simulink model "controlGPI_pos_2dof_sinMI"  (R2023b)
settings: Solver=ode45  StartTime=0.0  StopTime=tsim  FixedStep=5e-4  MaxStep=tstep
undefined symbols (not defined in the file): contr_robot_params, ddq, dq, ndof, NN_Bspline_params, NN_RBF_params, nn_select, Pc, q, q0, q_cero, q_eq, robot_params, t_qeq_init, t_tr_init, t_trtr, tau_L, tau_L_mags, tr_muestra, Wc, Zc
libraries: simulink x2
(part 1 of 2)
settings Model: Creator=HP  LastModifiedBy=HP

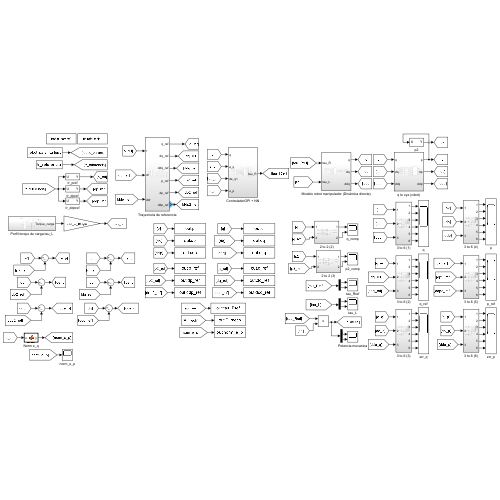
[thumbnail: Simulink's stored preview of the top-level diagram]
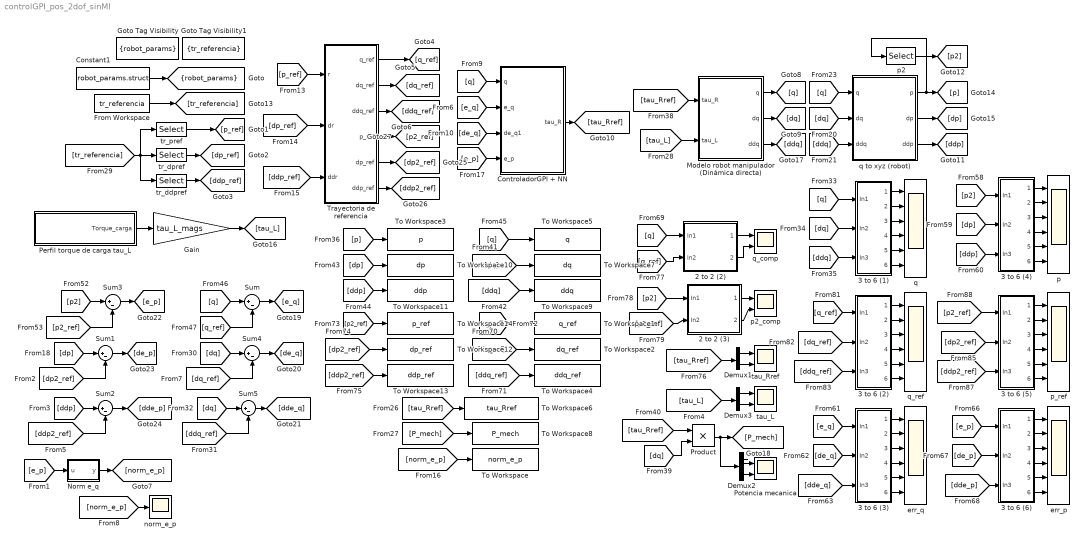
== system controlGPI_pos_2dof_sinMI ==
  2 to 2 (2) : Subsystem
  2 to 2 (3) : Subsystem
  3 to 6 (1) : Subsystem
  3 to 6 (2) : Subsystem
  3 to 6 (3) : Subsystem
  3 to 6 (4) : Subsystem
  3 to 6 (5) : Subsystem
  3 to 6 (6) : Subsystem
  Constant1 : Constant  Value=robot_params.struct  OutDataTypeStr=Bus: robot_params_bus
  ControladorGPI + NN : Subsystem
  Demux1 : Demux  Outputs=2
  Demux2 : Demux  Outputs=2
  Demux3 : Demux  Outputs=2
  From Workspace : FromWorkspace  VariableName=tr_referencia
  Gain : Gain  Gain=tau_L_mags
  Goto Tag Visibility : GotoTagVisibility  GotoTag=robot_params
  Goto Tag Visibility1 : GotoTagVisibility  GotoTag=tr_referencia
  Modelo robot manipulador (Dinámica directa) : Subsystem
  Norm e_q : MATLAB Function  TreatAsAtomicUnit=on
  Perfil torque de carga tau_L : Subsystem
  Potencia mecanica : Scope  NumInputPorts=2
  Product : Product
  Sum{,1..5} (6 alike) : Sum  Inputs=|+-
  To Workspace : ToWorkspace  VariableName=norm_e_p  SaveFormat=Timeseries  SampleTime=-1
  To Workspace1 : ToWorkspace  VariableName=q_ref  SaveFormat=Timeseries  SampleTime=-1
  To Workspace10 : ToWorkspace  VariableName=dp  SaveFormat=Timeseries  SampleTime=-1
  To Workspace11 : ToWorkspace  VariableName=ddp  SaveFormat=Timeseries  SampleTime=-1
  To Workspace12 : ToWorkspace  VariableName=dp_ref  SaveFormat=Timeseries  SampleTime=-1
  To Workspace13 : ToWorkspace  VariableName=ddp_ref  SaveFormat=Timeseries  SampleTime=-1
  To Workspace14 : ToWorkspace  VariableName=p_ref  SaveFormat=Timeseries  SampleTime=-1
  To Workspace2 : ToWorkspace  VariableName=dq_ref  SaveFormat=Timeseries  SampleTime=-1
  To Workspace3 : ToWorkspace  VariableName=p  SaveFormat=Timeseries  SampleTime=-1
  To Workspace4 : ToWorkspace  VariableName=ddq_ref  SaveFormat=Timeseries  SampleTime=-1
  To Workspace5 : ToWorkspace  VariableName=q  SaveFormat=Timeseries  SampleTime=-1
  To Workspace6 : ToWorkspace  VariableName=tau_Rref  SaveFormat=Timeseries  SampleTime=-1
  To Workspace7 : ToWorkspace  VariableName=dq  SaveFormat=Timeseries  SampleTime=-1
  To Workspace8 : ToWorkspace  VariableName=P_mech  SaveFormat=Timeseries  SampleTime=-1
  To Workspace9 : ToWorkspace  VariableName=ddq  SaveFormat=Timeseries  SampleTime=-1
  Trayectoria de referencia : Subsystem
  err_p : Scope  NumInputPorts=6
  err_q : Scope  NumInputPorts=6
  norm_e_p : Scope
  p : Scope  NumInputPorts=6
  p2 : Selector  NumberOfDimensions=2  InputPortWidth=3  IndexOptions=Index vector (dialog),Index vector (dialog)  Indices=[1:2],2  OutputSizes=1,1
  p2_comp : Scope  NumInputPorts=2
  p_ref : Scope  NumInputPorts=6
  q : Scope  NumInputPorts=6
  q to xyz (robot) : Subsystem
  q_comp : Scope  NumInputPorts=2
  q_ref : Scope  NumInputPorts=6
  tau_L : Scope  NumInputPorts=2
  tau_Rref : Scope  NumInputPorts=2
  tr_ddpref : Selector  NumberOfDimensions=2  InputPortWidth=3  IndexOptions=Index vector (dialog),Index vector (dialog)  Indices=[5:6],1  OutputSizes=1,1
  tr_dpref : Selector  NumberOfDimensions=2  InputPortWidth=3  IndexOptions=Index vector (dialog),Index vector (dialog)  Indices=[3:4],1  OutputSizes=1,1
  tr_pref : Selector  NumberOfDimensions=2  InputPortWidth=3  IndexOptions=Index vector (dialog),Index vector (dialog)  Indices=[1:2],1  OutputSizes=1,1
  tag scope: robot_params=scoped
  wires:
  From Workspace/1 -> [tr_referencia]
  Constant1/1 -> [robot_params]
  [tau_L] -> Modelo robot manipulador (Dinámica directa)/2(tau_L)
  [tau_Rref] -> Modelo robot manipulador (Dinámica directa)/1(tau_R)
  Modelo robot manipulador (Dinámica directa)/1(q) -> [q]
  Modelo robot manipulador (Dinámica directa)/2(dq) -> [dq]
  Modelo robot manipulador (Dinámica directa)/3(ddq) -> [ddq]
  ControladorGPI + NN/1(tau_R) -> [tau_Rref]
  [tr_referencia] -> tr_ddpref/1, tr_pref/1, tr_dpref/1
  tr_pref/1 -> [p_ref]
  tr_dpref/1 -> [dp_ref]
  tr_ddpref/1 -> [ddp_ref]
  [e_q] -> 3 to 6 (3)/1(In1)
  [dq_ref] -> 3 to 6 (2)/2(In2)
  [dq] -> 3 to 6 (1)/2(In2)
  2 to 2 (3)/1(1) -> p2_comp/1
  [tau_Rref] -> Product/1
  Product/1 -> Demux2/1, [P_mech]
  [q] -> 3 to 6 (1)/1(In1)
  [p2] -> 2 to 2 (3)/1(In1)
  [ddq_ref] -> 3 to 6 (2)/3(In3)
  3 to 6 (1)/5(Out5) -> q/5
  Demux2/1 -> Potencia mecanica/1
  [dde_p] -> 3 to 6 (6)/3(In3)
  [p2] -> 3 to 6 (4)/1(In1)
  Demux2/2 -> Potencia mecanica/2
  Demux1/2 -> tau_Rref/2
  3 to 6 (1)/6(Out6) -> q/6
  [de_q] -> 3 to 6 (3)/2(In2)
  [e_p] -> 3 to 6 (6)/1(In1)
  [dq] -> Product/2
  3 to 6 (1)/1(Out1) -> q/1
  [de_p] -> 3 to 6 (6)/2(In2)
  3 to 6 (1)/2(Out2) -> q/2
  [q_ref] -> 2 to 2 (2)/2(In2)
  [tau_Rref] -> Demux1/1
  [ddq] -> 3 to 6 (1)/3(In3)
  [p2_ref] -> 2 to 2 (3)/2(In2)
  [dde_q] -> 3 to 6 (3)/3(In3)
  3 to 6 (1)/4(Out4) -> q/4
  [q_ref] -> 3 to 6 (2)/1(In1)
  [ddp] -> 3 to 6 (4)/3(In3)
  [dp] -> 3 to 6 (4)/2(In2)
  Demux1/1 -> tau_Rref/1
  3 to 6 (1)/3(Out3) -> q/3
  q to xyz (robot)/1(p) -> [p], p2/1
  [dq] -> q to xyz (robot)/2(dq)
  [ddq] -> q to xyz (robot)/3(ddq)
  [q] -> To Workspace5/1
  [tau_Rref] -> To Workspace6/1
  [dq_ref] -> To Workspace2/1
  [q] -> q to xyz (robot)/1(q)
  [ddq] -> To Workspace9/1
  [p2_ref] -> To Workspace14/1
  [ddq_ref] -> To Workspace4/1
  [q_ref] -> To Workspace1/1
  q to xyz (robot)/2(dp) -> [dp]
  [dp] -> To Workspace10/1
  [dp2_ref] -> To Workspace12/1
  q to xyz (robot)/3(ddp) -> [ddp]
  [P_mech] -> To Workspace8/1
  [ddp] -> To Workspace11/1
  [p] -> To Workspace3/1
  [dq] -> To Workspace7/1
  p2/1 -> [p2]
  [ddp2_ref] -> To Workspace13/1
  2 to 2 (2)/1(1) -> q_comp/1
  2 to 2 (2)/2(2) -> q_comp/2
  3 to 6 (2)/4(Out4) -> q_ref/4
  3 to 6 (2)/6(Out6) -> q_ref/6
  3 to 6 (2)/3(Out3) -> q_ref/3
  3 to 6 (2)/1(Out1) -> q_ref/1
  3 to 6 (2)/2(Out2) -> q_ref/2
  3 to 6 (2)/5(Out5) -> q_ref/5
  3 to 6 (3)/4(Out4) -> err_q/4
  3 to 6 (3)/6(Out6) -> err_q/6
  3 to 6 (3)/3(Out3) -> err_q/3
  3 to 6 (3)/1(Out1) -> err_q/1
  3 to 6 (3)/2(Out2) -> err_q/2
  3 to 6 (3)/5(Out5) -> err_q/5
  3 to 6 (4)/4(Out4) -> p/4
  3 to 6 (4)/6(Out6) -> p/6
  3 to 6 (4)/3(Out3) -> p/3
  3 to 6 (4)/1(Out1) -> p/1
  3 to 6 (4)/2(Out2) -> p/2
  3 to 6 (4)/5(Out5) -> p/5
  3 to 6 (5)/4(Out4) -> p_ref/4
  3 to 6 (5)/6(Out6) -> p_ref/6
  3 to 6 (5)/3(Out3) -> p_ref/3
  3 to 6 (5)/1(Out1) -> p_ref/1
  3 to 6 (5)/2(Out2) -> p_ref/2
  3 to 6 (5)/5(Out5) -> p_ref/5
  [p2_ref] -> 3 to 6 (5)/1(In1)
  [dp2_ref] -> 3 to 6 (5)/2(In2)
  [ddp2_ref] -> 3 to 6 (5)/3(In3)
  3 to 6 (6)/4(Out4) -> err_p/4
  3 to 6 (6)/6(Out6) -> err_p/6
  3 to 6 (6)/3(Out3) -> err_p/3
  3 to 6 (6)/1(Out1) -> err_p/1
  3 to 6 (6)/2(Out2) -> err_p/2
  3 to 6 (6)/5(Out5) -> err_p/5
  2 to 2 (3)/2(2) -> p2_comp/2
  [norm_e_p] -> To Workspace/1
  [e_p] -> ControladorGPI + NN/4(e_p)
  [q] -> 2 to 2 (2)/1(In1)
  [e_q] -> ControladorGPI + NN/2(e_q)
  Demux3/2 -> tau_L/2
  Demux3/1 -> tau_L/1
  [tau_L] -> Demux3/1
  [q] -> ControladorGPI + NN/1(q)
  [de_q] -> ControladorGPI + NN/3(de_q1)
  Trayectoria de referencia/6(ddp_ref) -> [ddp2_ref]
  Trayectoria de referencia/5(dp_ref) -> [dp2_ref]
  Trayectoria de referencia/1(q_ref) -> [q_ref]
  [dp_ref] -> Trayectoria de referencia/2(dr)
  Trayectoria de referencia/3(ddq_ref) -> [ddq_ref]
  Trayectoria de referencia/2(dq_ref) -> [dq_ref]
  [p_ref] -> Trayectoria de referencia/1(r)
  [ddp_ref] -> Trayectoria de referencia/3(ddr)
  Trayectoria de referencia/4(p_ref) -> [p2_ref]
  [ddq_ref] -> Sum5/2
  [ddp] -> Sum2/1
  [ddp2_ref] -> Sum2/2
  Sum4/1 -> [de_q]
  [dq] -> Sum4/1
  [dq_ref] -> Sum4/2
  [dp] -> Sum1/1
  [dp2_ref] -> Sum1/2
  [q] -> Sum/1
  [dq] -> Sum5/1
  [p2_ref] -> Sum3/2
  [norm_e_p] -> norm_e_p/1
  Sum3/1 -> [e_p]
  [e_p] -> Norm e_q/1(u)
  Sum/1 -> [e_q]
  [p2] -> Sum3/1
  Sum2/1 -> [dde_p]
  Sum5/1 -> [dde_q]
  Sum1/1 -> [de_p]
  Norm e_q/1(y) -> [norm_e_p]
  [q_ref] -> Sum/2
  Perfil torque de carga tau_L/1(Torque_carga) -> Gain/1
  Gain/1 -> [tau_L]

== system controlGPI_pos_2dof_sinMI/2 to 2 (2) ==
  In1 : Inport
  In2 : Inport  Port=2
  Demux3 : Demux  Outputs=2
  Demux4 : Demux  Outputs=2
  Mux8 : Mux  Inputs=2
  Mux9 : Mux  Inputs=2
  1 : Outport
  2 : Outport  Port=2
  wires:
  Demux3/1 -> Mux8/1
  Demux3/2 -> Mux9/1
  Mux9/1 -> 2/1
  Demux4/2 -> Mux9/2
  Demux4/1 -> Mux8/2
  Mux8/1 -> 1/1
  In1/1 -> Demux3/1
  In2/1 -> Demux4/1

== system controlGPI_pos_2dof_sinMI/2 to 2 (3) ==
  In1 : Inport
  In2 : Inport  Port=2
  Demux3 : Demux  Outputs=2
  Demux4 : Demux  Outputs=2
  Mux8 : Mux  Inputs=2
  Mux9 : Mux  Inputs=2
  1 : Outport
  2 : Outport  Port=2
  wires:
  Demux3/1 -> Mux8/1
  Demux3/2 -> Mux9/1
  Mux9/1 -> 2/1
  Demux4/2 -> Mux9/2
  Demux4/1 -> Mux8/2
  Mux8/1 -> 1/1
  In1/1 -> Demux3/1
  In2/1 -> Demux4/1

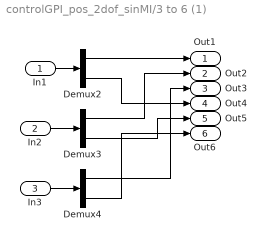
== system controlGPI_pos_2dof_sinMI/3 to 6 (1) ==
  In1 : Inport
  In2 : Inport  Port=2
  In3 : Inport  Port=3
  Demux2 : Demux  Outputs=2
  Demux3 : Demux  Outputs=2
  Demux4 : Demux  Outputs=2
  Out1 : Outport
  Out2 : Outport  Port=2
  Out3 : Outport  Port=3
  Out4 : Outport  Port=4
  Out5 : Outport  Port=5
  Out6 : Outport  Port=6
  wires:
  In3/1 -> Demux4/1
  Demux4/1 -> Out3/1
  Demux2/1 -> Out1/1
  Demux3/2 -> Out5/1
  Demux3/1 -> Out2/1
  In1/1 -> Demux2/1
  Demux4/2 -> Out6/1
  Demux2/2 -> Out4/1
  In2/1 -> Demux3/1

== system controlGPI_pos_2dof_sinMI/3 to 6 (2) ==
  In1 : Inport
  In2 : Inport  Port=2
  In3 : Inport  Port=3
  Demux2 : Demux  Outputs=2
  Demux3 : Demux  Outputs=2
  Demux4 : Demux  Outputs=2
  Out1 : Outport
  Out2 : Outport  Port=2
  Out3 : Outport  Port=3
  Out4 : Outport  Port=4
  Out5 : Outport  Port=5
  Out6 : Outport  Port=6
  wires:
  In3/1 -> Demux4/1
  Demux4/1 -> Out3/1
  Demux2/1 -> Out1/1
  Demux3/2 -> Out5/1
  Demux3/1 -> Out2/1
  In1/1 -> Demux2/1
  Demux4/2 -> Out6/1
  Demux2/2 -> Out4/1
  In2/1 -> Demux3/1

== system controlGPI_pos_2dof_sinMI/3 to 6 (3) ==
  In1 : Inport
  In2 : Inport  Port=2
  In3 : Inport  Port=3
  Demux2 : Demux  Outputs=2
  Demux3 : Demux  Outputs=2
  Demux4 : Demux  Outputs=2
  Out1 : Outport
  Out2 : Outport  Port=2
  Out3 : Outport  Port=3
  Out4 : Outport  Port=4
  Out5 : Outport  Port=5
  Out6 : Outport  Port=6
  wires:
  In3/1 -> Demux4/1
  Demux4/1 -> Out3/1
  Demux2/1 -> Out1/1
  Demux3/2 -> Out5/1
  Demux3/1 -> Out2/1
  In1/1 -> Demux2/1
  Demux4/2 -> Out6/1
  Demux2/2 -> Out4/1
  In2/1 -> Demux3/1

== system controlGPI_pos_2dof_sinMI/3 to 6 (4) ==
  In1 : Inport
  In2 : Inport  Port=2
  In3 : Inport  Port=3
  Demux2 : Demux  Outputs=2
  Demux3 : Demux  Outputs=2
  Demux4 : Demux  Outputs=2
  Out1 : Outport
  Out2 : Outport  Port=2
  Out3 : Outport  Port=3
  Out4 : Outport  Port=4
  Out5 : Outport  Port=5
  Out6 : Outport  Port=6
  wires:
  In3/1 -> Demux4/1
  Demux4/1 -> Out3/1
  Demux2/1 -> Out1/1
  Demux3/2 -> Out5/1
  Demux3/1 -> Out2/1
  In1/1 -> Demux2/1
  Demux4/2 -> Out6/1
  Demux2/2 -> Out4/1
  In2/1 -> Demux3/1

== system controlGPI_pos_2dof_sinMI/3 to 6 (5) ==
  In1 : Inport
  In2 : Inport  Port=2
  In3 : Inport  Port=3
  Demux2 : Demux  Outputs=2
  Demux3 : Demux  Outputs=2
  Demux4 : Demux  Outputs=2
  Out1 : Outport
  Out2 : Outport  Port=2
  Out3 : Outport  Port=3
  Out4 : Outport  Port=4
  Out5 : Outport  Port=5
  Out6 : Outport  Port=6
  wires:
  In3/1 -> Demux4/1
  Demux4/1 -> Out3/1
  Demux2/1 -> Out1/1
  Demux3/2 -> Out5/1
  Demux3/1 -> Out2/1
  In1/1 -> Demux2/1
  Demux4/2 -> Out6/1
  Demux2/2 -> Out4/1
  In2/1 -> Demux3/1

== system controlGPI_pos_2dof_sinMI/3 to 6 (6) ==
  In1 : Inport
  In2 : Inport  Port=2
  In3 : Inport  Port=3
  Demux2 : Demux  Outputs=2
  Demux3 : Demux  Outputs=2
  Demux4 : Demux  Outputs=2
  Out1 : Outport
  Out2 : Outport  Port=2
  Out3 : Outport  Port=3
  Out4 : Outport  Port=4
  Out5 : Outport  Port=5
  Out6 : Outport  Port=6
  wires:
  In3/1 -> Demux4/1
  Demux4/1 -> Out3/1
  Demux2/1 -> Out1/1
  Demux3/2 -> Out5/1
  Demux3/1 -> Out2/1
  In1/1 -> Demux2/1
  Demux4/2 -> Out6/1
  Demux2/2 -> Out4/1
  In2/1 -> Demux3/1

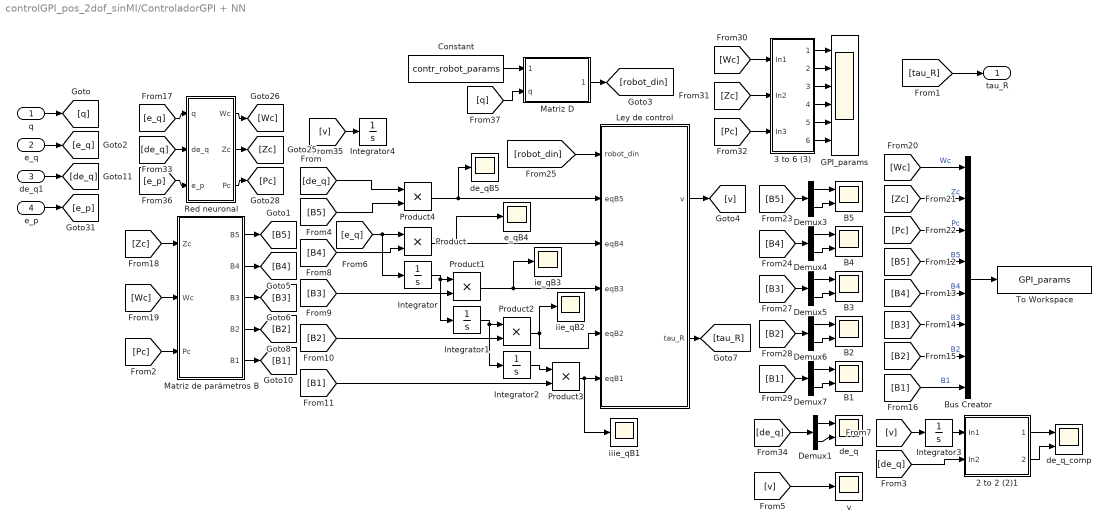
== system controlGPI_pos_2dof_sinMI/ControladorGPI + NN ==
  q : Inport
  e_q : Inport  Port=2
  de_q1 : Inport  Port=3
  e_p : Inport  Port=4
  2 to 2 (2)1 : Subsystem
  3 to 6 (3) : Subsystem
  B{1..5} (5 alike) : Scope  NumInputPorts=2
  Bus Creator : BusCreator  Inputs=8
  Constant : Constant  Value=contr_robot_params  OutDataTypeStr=Bus: robot_params_bus
  Demux{1,3..7} (6 alike) : Demux  Outputs=2
  GPI_params : Scope  NumInputPorts=6
  Integrator{,1..4} (5 alike) : Integrator
  Ley de control : MATLAB Function  TreatAsAtomicUnit=on
  Matriz D : MATLAB Function  TreatAsAtomicUnit=on
  Matriz de parámetros B : MATLAB Function  TreatAsAtomicUnit=on
  Product{,1..4} (5 alike) : Product
  Red neuronal : Subsystem
  To Workspace : ToWorkspace  VariableName=GPI_params  SaveFormat=Timeseries  SampleTime=-1
  de_q : Scope  NumInputPorts=2
  de_qB5 : Scope
  de_q_comp : Scope  NumInputPorts=2
  e_qB4 : Scope
  ie_qB3 : Scope
  iie_qB2 : Scope
  iiie_qB1 : Scope
  v : Scope
  tau_R : Outport
  wires:
  Ley de control/2(tau_R) -> [tau_R]
  [tau_R] -> tau_R/1
  e_q/1 -> [e_q]
  [e_q] -> Integrator/1, Product/1
  Integrator/1 -> Integrator1/1, Product1/1
  Integrator1/1 -> Integrator2/1, Product2/1
  Integrator2/1 -> Product3/1
  Product3/1 -> iiie_qB1/1, Ley de control/6(eqB1)
  Product2/1 -> iie_qB2/1, Ley de control/5(eqB2)
  Product1/1 -> ie_qB3/1, Ley de control/4(eqB3)
  Product/1 -> e_qB4/1, Ley de control/3(eqB4)
  Ley de control/1(v) -> [v]
  Product4/1 -> de_qB5/1, Ley de control/2(eqB5)
  [Zc] -> Matriz de parámetros B/1(Zc)
  [Wc] -> Matriz de parámetros B/2(Wc)
  [Pc] -> Matriz de parámetros B/3(Pc)
  Matriz de parámetros B/1(B5) -> [B5]
  Matriz de parámetros B/2(B4) -> [B4]
  Matriz de parámetros B/3(B3) -> [B3]
  Matriz de parámetros B/4(B2) -> [B2]
  Matriz de parámetros B/5(B1) -> [B1]
  [B5] -> Product4/2
  [B4] -> Product/2
  [B3] -> Product1/2
  [B2] -> Product2/2
  [B1] -> Product3/2
  Bus Creator/1 -> To Workspace/1
  [Wc] -> Bus Creator/1  "Wc"
  [Zc] -> Bus Creator/2  "Zc"
  [Pc] -> Bus Creator/3  "Pc"
  [B5] -> Bus Creator/4  "B5"
  [B4] -> Bus Creator/5  "B4"
  [B3] -> Bus Creator/6  "B3"
  [B2] -> Bus Creator/7  "B2"
  [B1] -> Bus Creator/8  "B1"
  Demux3/2 -> B5/2
  Demux3/1 -> B5/1
  [B5] -> Demux3/1
  Demux4/2 -> B4/2
  Demux4/1 -> B4/1
  [B4] -> Demux4/1
  Demux5/1 -> B3/1
  Demux5/2 -> B3/2
  [B3] -> Demux5/1
  Demux6/1 -> B2/1
  Demux6/2 -> B2/2
  [B2] -> Demux6/1
  Demux7/1 -> B1/1
  Demux7/2 -> B1/2
  [B1] -> Demux7/1
  Red neuronal/2(Zc) -> [Zc]
  Red neuronal/1(Wc) -> [Wc]
  Red neuronal/3(Pc) -> [Pc]
  [de_q] -> Red neuronal/2(de_q)
  [Wc] -> 3 to 6 (3)/1(In1)
  [Zc] -> 3 to 6 (3)/2(In2)
  [Pc] -> 3 to 6 (3)/3(In3)
  3 to 6 (3)/4(Out4) -> GPI_params/4
  3 to 6 (3)/2(Out2) -> GPI_params/2
  3 to 6 (3)/3(Out3) -> GPI_params/3
  3 to 6 (3)/5(Out5) -> GPI_params/5
  3 to 6 (3)/1(Out1) -> GPI_params/1
  3 to 6 (3)/6(Out6) -> GPI_params/6
  [e_q] -> Red neuronal/1(q)
  [de_q] -> Demux1/1
  Demux1/1 -> de_q/1
  Demux1/2 -> de_q/2
  de_q1/1 -> [de_q]
  e_p/1 -> [e_p]
  [e_p] -> Red neuronal/3(e_p)
  [robot_din] -> Ley de control/1(robot_din)
  q/1 -> [q]
  [v] -> Integrator3/1
  Integrator3/1 -> 2 to 2 (2)1/1(In1)
  [de_q] -> 2 to 2 (2)1/2(In2)
  2 to 2 (2)1/1(1) -> de_q_comp/1
  2 to 2 (2)1/2(2) -> de_q_comp/2
  [v] -> v/1
  [v] -> Integrator4/1
  [de_q] -> Product4/1
  Constant/1 -> Matriz D/1(robot_params)
  [q] -> Matriz D/2(q)
  Matriz D/1(robot_din) -> [robot_din]

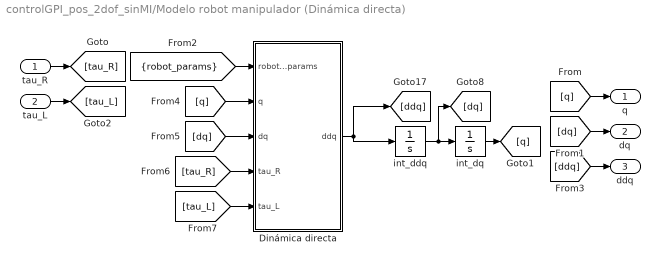
== system controlGPI_pos_2dof_sinMI/Modelo robot manipulador (Dinámica directa) ==
  tau_R : Inport
  tau_L : Inport  Port=2
  Dinámica directa : MATLAB Function  TreatAsAtomicUnit=on
  int_ddq : Integrator  InitialCondition=q_cero
  int_dq : Integrator  InitialCondition=q_eq
  q : Outport
  dq : Outport  Port=2
  ddq : Outport  Port=3
  wires:
  [tau_L] -> Dinámica directa/5(tau_L)
  int_ddq/1 -> [dq], int_dq/1
  [robot_params] -> Dinámica directa/1(robot_params)
  [dq] -> Dinámica directa/3(dq)
  int_dq/1 -> [q]
  [tau_R] -> Dinámica directa/4(tau_R)
  Dinámica directa/1(ddq) -> int_ddq/1, [ddq]
  [q] -> q/1
  [dq] -> dq/1
  [ddq] -> ddq/1
  tau_R/1 -> [tau_R]
  tau_L/1 -> [tau_L]
  [q] -> Dinámica directa/2(q)

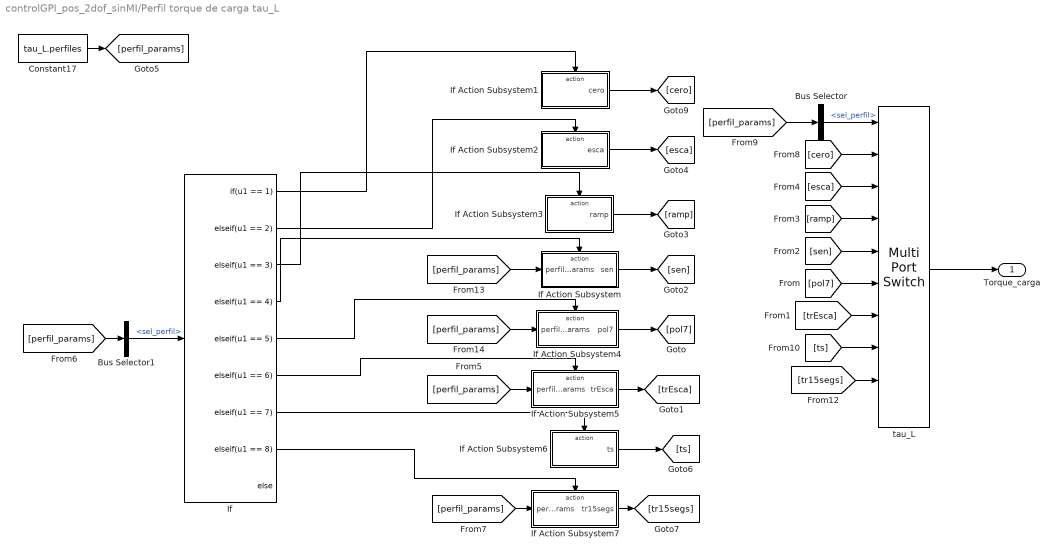
== system controlGPI_pos_2dof_sinMI/Perfil torque de carga tau_L ==
  Bus Selector : BusSelector  OutputSignals=sel_perfil
  Bus Selector1 : BusSelector  OutputSignals=sel_perfil
  Constant17 : Constant  Value=tau_L.perfiles  OutDataTypeStr=Bus: Perfil_bus
  If : If  IfExpression=u1 == 1  ElseIfExpressions=u1 == 2,u1 == 3,u1 == 4,u1 == 5,u1 == 6,u1 == 7,u1 == 8
  If Action Subsystem : Subsystem  TreatAsAtomicUnit=on
  If Action Subsystem1 : Subsystem  TreatAsAtomicUnit=on
  If Action Subsystem2 : Subsystem  TreatAsAtomicUnit=on
  If Action Subsystem3 : Subsystem  TreatAsAtomicUnit=on
  If Action Subsystem4 : Subsystem  TreatAsAtomicUnit=on
  If Action Subsystem5 : Subsystem  TreatAsAtomicUnit=on
  If Action Subsystem6 : Subsystem  TreatAsAtomicUnit=on
  If Action Subsystem7 : Subsystem  TreatAsAtomicUnit=on
  tau_L : MultiPortSwitch  Inputs=9  SaturateOnIntegerOverflow=off  InputSameDT=off
  Torque_carga : Outport
  wires:
  tau_L/1 -> Torque_carga/1
  [ramp] -> tau_L/4
  [trEsca] -> tau_L/7
  [pol7] -> tau_L/6
  [sen] -> tau_L/5
  [esca] -> tau_L/3
  Constant17/1 -> [perfil_params]
  [ts] -> tau_L/8
  [tr15segs] -> tau_L/9
  Bus Selector/1 -> tau_L/1  "<sel_perfil>"
  [perfil_params] -> Bus Selector/1
  If Action Subsystem/1(sen) -> [sen]
  [perfil_params] -> Bus Selector1/1
  Bus Selector1/1 -> If/1  "<sel_perfil>"
  If/4 -> If Action Subsystem/Action
  If Action Subsystem1/1(cero) -> [cero]
  [cero] -> tau_L/2
  [perfil_params] -> If Action Subsystem/1(perfil_params)
  If/1 -> If Action Subsystem1/Action
  If Action Subsystem2/1(esca) -> [esca]
  If/2 -> If Action Subsystem2/Action
  If Action Subsystem3/1(ramp) -> [ramp]
  If/3 -> If Action Subsystem3/Action
  [perfil_params] -> If Action Subsystem4/1(perfil_params)
  If/5 -> If Action Subsystem4/Action
  If Action Subsystem4/1(pol7) -> [pol7]
  If Action Subsystem5/1(trEsca) -> [trEsca]
  [perfil_params] -> If Action Subsystem5/1(perfil_params)
  If Action Subsystem6/1(ts) -> [ts]
  If/6 -> If Action Subsystem5/Action
  If/7 -> If Action Subsystem6/Action
  If Action Subsystem7/1(tr15segs) -> [tr15segs]
  If/8 -> If Action Subsystem7/Action
  [perfil_params] -> If Action Subsystem7/1(perfil_params)

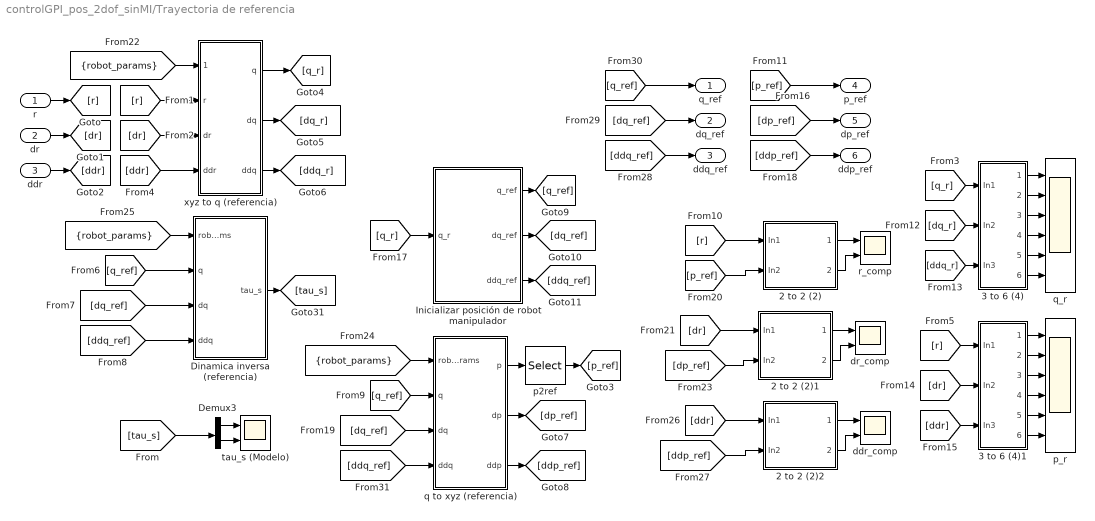
== system controlGPI_pos_2dof_sinMI/Trayectoria de referencia ==
  r : Inport
  dr : Inport  Port=2
  ddr : Inport  Port=3
  2 to 2 (2) : Subsystem
  2 to 2 (2)1 : Subsystem
  2 to 2 (2)2 : Subsystem
  3 to 6 (4) : Subsystem
  3 to 6 (4)1 : Subsystem
  Demux3 : Demux  Outputs=2
  Dinamica inversa (referencia) : MATLAB Function  TreatAsAtomicUnit=on
  Inicializar posición de robot manipulador : Subsystem
  ddr_comp : Scope  NumInputPorts=2
  dr_comp : Scope  NumInputPorts=2
  p2ref : Selector  NumberOfDimensions=2  InputPortWidth=3  IndexOptions=Index vector (dialog),Index vector (dialog)  Indices=[1:2],2  OutputSizes=1,1
  p_r : Scope  NumInputPorts=6
  q to xyz (referencia) : MATLAB Function  TreatAsAtomicUnit=on
  q_r : Scope  NumInputPorts=6
  r_comp : Scope  NumInputPorts=2
  tau_s (Modelo) : Scope  NumInputPorts=2
  xyz to q (referencia) : MATLAB Function  TreatAsAtomicUnit=on
  q_ref : Outport
  dq_ref : Outport  Port=2
  ddq_ref : Outport  Port=3
  p_ref : Outport  Port=4
  dp_ref : Outport  Port=5
  ddp_ref : Outport  Port=6
  wires:
  xyz to q (referencia)/1(q) -> [q_r]
  [robot_params] -> xyz to q (referencia)/1(robot_params)
  [dq_ref] -> Dinamica inversa (referencia)/3(dq)
  [q_ref] -> Dinamica inversa (referencia)/2(q)
  [q_ref] -> q to xyz (referencia)/2(q)
  [r] -> xyz to q (referencia)/2(r)
  xyz to q (referencia)/2(dq) -> [dq_r]
  q to xyz (referencia)/1(p) -> p2ref/1
  [robot_params] -> Dinamica inversa (referencia)/1(robot_params)
  Dinamica inversa (referencia)/1(tau_s) -> [tau_s]
  xyz to q (referencia)/3(ddq) -> [ddq_r]
  [ddq_ref] -> Dinamica inversa (referencia)/4(ddq)
  [ddr] -> xyz to q (referencia)/4(ddr)
  [dr] -> xyz to q (referencia)/3(dr)
  r/1 -> [r]
  dr/1 -> [dr]
  ddr/1 -> [ddr]
  [tau_s] -> Demux3/1
  [q_r] -> Inicializar posición de robot manipulador/1(q_r)
  [robot_params] -> q to xyz (referencia)/1(robot_params)
  p2ref/1 -> [p_ref]
  [r] -> 2 to 2 (2)/1(In1)
  [p_ref] -> p_ref/1
  [dp_ref] -> dp_ref/1
  [ddp_ref] -> ddp_ref/1
  [p_ref] -> 2 to 2 (2)/2(In2)
  [dp_ref] -> 2 to 2 (2)1/2(In2)
  [dr] -> 2 to 2 (2)1/1(In1)
  [ddp_ref] -> 2 to 2 (2)2/2(In2)
  [ddr] -> 2 to 2 (2)2/1(In1)
  Inicializar posición de robot manipulador/1(q_ref) -> [q_ref]
  Inicializar posición de robot manipulador/2(dq_ref) -> [dq_ref]
  Inicializar posición de robot manipulador/3(ddq_ref) -> [ddq_ref]
  [ddq_ref] -> ddq_ref/1
  [dq_ref] -> dq_ref/1
  [q_ref] -> q_ref/1
  [ddr] -> 3 to 6 (4)1/3(In3)
  [dq_r] -> 3 to 6 (4)/2(In2)
  [r] -> 3 to 6 (4)1/1(In1)
  [q_r] -> 3 to 6 (4)/1(In1)
  [dr] -> 3 to 6 (4)1/2(In2)
  [ddq_r] -> 3 to 6 (4)/3(In3)
  2 to 2 (2)/1(1) -> r_comp/1
  2 to 2 (2)/2(2) -> r_comp/2
  2 to 2 (2)1/1(1) -> dr_comp/1
  2 to 2 (2)1/2(2) -> dr_comp/2
  2 to 2 (2)2/1(1) -> ddr_comp/1
  2 to 2 (2)2/2(2) -> ddr_comp/2
  3 to 6 (4)/1(Out1) -> q_r/1
  3 to 6 (4)/6(Out6) -> q_r/6
  3 to 6 (4)/5(Out5) -> q_r/5
  3 to 6 (4)/2(Out2) -> q_r/2
  3 to 6 (4)/3(Out3) -> q_r/3
  3 to 6 (4)/4(Out4) -> q_r/4
  3 to 6 (4)1/1(Out1) -> p_r/1
  3 to 6 (4)1/6(Out6) -> p_r/6
  3 to 6 (4)1/5(Out5) -> p_r/5
  3 to 6 (4)1/2(Out2) -> p_r/2
  3 to 6 (4)1/3(Out3) -> p_r/3
  3 to 6 (4)1/4(Out4) -> p_r/4
  Demux3/1 -> tau_s (Modelo)/1
  Demux3/2 -> tau_s (Modelo)/2
  [dq_ref] -> q to xyz (referencia)/3(dq)
  [ddq_ref] -> q to xyz (referencia)/4(ddq)
  q to xyz (referencia)/2(dp) -> [dp_ref]
  q to xyz (referencia)/3(ddp) -> [ddp_ref]

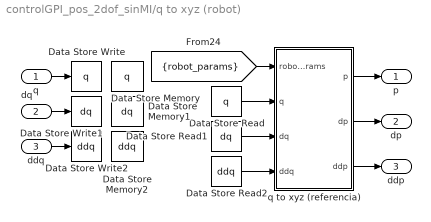
== system controlGPI_pos_2dof_sinMI/q to xyz (robot) ==
  q : Inport
  dq : Inport  Port=2
  ddq : Inport  Port=3
  Data Store Memory : DataStoreMemory  DataStoreName=q  WriteAfterWriteMsg=warning  InitialValue=zeros(size(q(:,1)))  ShowAdditionalParam=off
  Data Store Memory1 : DataStoreMemory  DataStoreName=dq  WriteAfterWriteMsg=warning  InitialValue=zeros(size(dq(:,1)))  ShowAdditionalParam=off
  Data Store Memory2 : DataStoreMemory  DataStoreName=ddq  WriteAfterWriteMsg=warning  InitialValue=zeros(size(ddq(:,1)))  ShowAdditionalParam=off
  Data Store Read : DataStoreRead  DataStoreName=q  IndexOptions=Index vector (dialog)  Indices=1  OutputSizes=1
  Data Store Read1 : DataStoreRead  DataStoreName=dq  IndexOptions=Index vector (dialog)  Indices=1  OutputSizes=1
  Data Store Read2 : DataStoreRead  DataStoreName=ddq  IndexOptions=Index vector (dialog)  Indices=1  OutputSizes=1
  Data Store Write : DataStoreWrite  DataStoreName=q  IndexOptions=Index vector (dialog)  Indices=1  OutputSizes=1
  Data Store Write1 : DataStoreWrite  DataStoreName=dq  IndexOptions=Index vector (dialog)  Indices=1  OutputSizes=1
  Data Store Write2 : DataStoreWrite  DataStoreName=ddq  IndexOptions=Index vector (dialog)  Indices=1  OutputSizes=1
  q to xyz (referencia) : MATLAB Function  TreatAsAtomicUnit=on
  p : Outport
  dp : Outport  Port=2
  ddp : Outport  Port=3
  wires:
  q/1 -> Data Store Write/1
  ddq/1 -> Data Store Write2/1
  dq/1 -> Data Store Write1/1
  Data Store Read/1 -> q to xyz (referencia)/2(q)
  Data Store Read1/1 -> q to xyz (referencia)/3(dq)
  Data Store Read2/1 -> q to xyz (referencia)/4(ddq)
  q to xyz (referencia)/1(p) -> p/1
  q to xyz (referencia)/2(dp) -> dp/1
  q to xyz (referencia)/3(ddp) -> ddp/1
  [robot_params] -> q to xyz (referencia)/1(robot_params)

== system controlGPI_pos_2dof_sinMI/ControladorGPI + NN/2 to 2 (2)1 ==
  In1 : Inport
  In2 : Inport  Port=2
  Demux3 : Demux  Outputs=2
  Demux4 : Demux  Outputs=2
  Mux8 : Mux  Inputs=2
  Mux9 : Mux  Inputs=2
  1 : Outport
  2 : Outport  Port=2
  wires:
  Demux3/1 -> Mux8/1
  Demux3/2 -> Mux9/1
  Mux9/1 -> 2/1
  Demux4/2 -> Mux9/2
  Demux4/1 -> Mux8/2
  Mux8/1 -> 1/1
  In1/1 -> Demux3/1
  In2/1 -> Demux4/1

== system controlGPI_pos_2dof_sinMI/ControladorGPI + NN/3 to 6 (3) ==
  In1 : Inport
  In2 : Inport  Port=2
  In3 : Inport  Port=3
  Demux2 : Demux  Outputs=2
  Demux3 : Demux  Outputs=2
  Demux4 : Demux  Outputs=2
  Out1 : Outport
  Out2 : Outport  Port=2
  Out3 : Outport  Port=3
  Out4 : Outport  Port=4
  Out5 : Outport  Port=5
  Out6 : Outport  Port=6
  wires:
  In3/1 -> Demux4/1
  Demux4/1 -> Out3/1
  Demux2/1 -> Out1/1
  Demux3/2 -> Out5/1
  Demux3/1 -> Out2/1
  In1/1 -> Demux2/1
  Demux4/2 -> Out6/1
  Demux2/2 -> Out4/1
  In2/1 -> Demux3/1

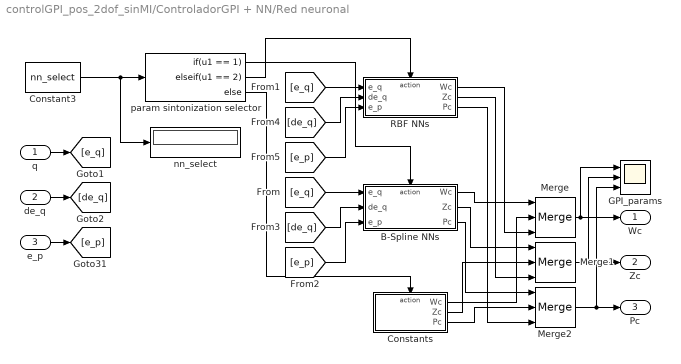
== system controlGPI_pos_2dof_sinMI/ControladorGPI + NN/Red neuronal ==
  q : Inport
  de_q : Inport  Port=2
  e_p : Inport  Port=3
  B-Spline NNs : Subsystem  TreatAsAtomicUnit=on
  Constant3 : Constant  Value=nn_select
  Constants : Subsystem  TreatAsAtomicUnit=on
  GPI_params : Scope  NumInputPorts=3
  Merge : Merge  Inputs=3
  Merge1 : Merge  Inputs=3
  Merge2 : Merge  Inputs=3
  RBF NNs : Subsystem  TreatAsAtomicUnit=on
  nn_select : Display
  param sintonization selector : If  IfExpression=u1 == 1  ElseIfExpressions=u1 == 2
  Wc : Outport
  Zc : Outport  Port=2
  Pc : Outport  Port=3
  wires:
  param sintonization selector/1 -> B-Spline NNs/Action
  B-Spline NNs/1(Wc) -> Merge/1
  param sintonization selector/3 -> Constants/Action
  Constant3/1 -> nn_select/1, param sintonization selector/1
  B-Spline NNs/2(Zc) -> Merge1/1
  B-Spline NNs/3(Pc) -> Merge2/1
  Constants/1(Wc) -> Merge/2
  Constants/2(Zc) -> Merge1/2
  Constants/3(Pc) -> Merge2/2
  q/1 -> [e_q]
  de_q/1 -> [de_q]
  param sintonization selector/2 -> RBF NNs/Action
  RBF NNs/2(Zc) -> Merge1/3
  RBF NNs/1(Wc) -> Merge/3
  RBF NNs/3(Pc) -> Merge2/3
  Merge/1 -> GPI_params/1, Wc/1
  Merge1/1 -> GPI_params/2, Zc/1
  Merge2/1 -> GPI_params/3, Pc/1
  [e_q] -> B-Spline NNs/1(e_q)
  [de_q] -> B-Spline NNs/2(de_q)
  [e_q] -> RBF NNs/1(e_q)
  [de_q] -> RBF NNs/2(de_q)
  e_p/1 -> [e_p]
  [e_p] -> RBF NNs/3(e_p)
  [e_p] -> B-Spline NNs/3(e_p)

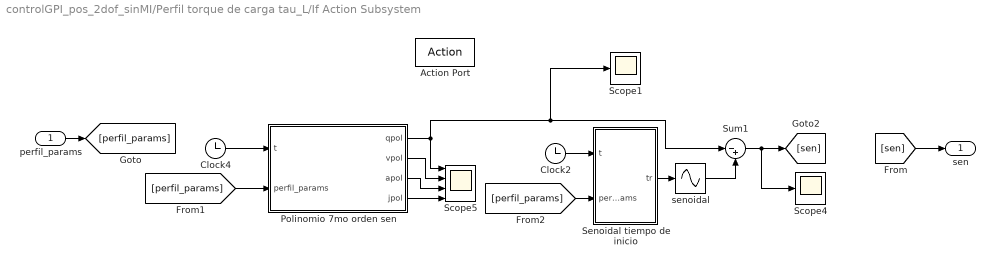
== system controlGPI_pos_2dof_sinMI/Perfil torque de carga tau_L/If Action Subsystem ==
  perfil_params : Inport
  Action Port : ActionPort
  Clock2 : Clock
  Clock4 : Clock
  Polinomio 7mo orden sen : MATLAB Function  TreatAsAtomicUnit=on
  Scope1 : Scope
  Scope4 : Scope
  Scope5 : Scope  NumInputPorts=4
  Senoidal tiempo de inicio : MATLAB Function  TreatAsAtomicUnit=on
  Sum1 : Sum  Inputs=|-+
  senoidal : Sin  TimeSource=Use external signal  Frequency=6.2832  Phase=1.5708  SampleTime=0
  sen : Outport
  wires:
  Clock4/1 -> Polinomio 7mo orden sen/1(t)
  Polinomio 7mo orden sen/1(qpol) -> Scope1/1, Sum1/1, Scope5/1
  Sum1/1 -> Scope4/1, [sen]
  Polinomio 7mo orden sen/4(jpol) -> Scope5/4
  Polinomio 7mo orden sen/3(apol) -> Scope5/3
  Clock2/1 -> Senoidal tiempo de inicio/1(t)
  [perfil_params] -> Polinomio 7mo orden sen/2(perfil_params)
  Polinomio 7mo orden sen/2(vpol) -> Scope5/2
  senoidal/1 -> Sum1/2
  Senoidal tiempo de inicio/1(tr) -> senoidal/1
  [sen] -> sen/1
  perfil_params/1 -> [perfil_params]
  [perfil_params] -> Senoidal tiempo de inicio/2(perfil_params)

== system controlGPI_pos_2dof_sinMI/Perfil torque de carga tau_L/If Action Subsystem1 ==
  Action Port : ActionPort
  Constant : Constant  Value=0
  cero : Outport
  wires:
  Constant/1 -> cero/1

== system controlGPI_pos_2dof_sinMI/Perfil torque de carga tau_L/If Action Subsystem2 ==
  Action Port : ActionPort
  Scope3 : Scope
  Sum : Sum  Inputs=|++
  escalon1 : Step  Time=2.5  After=0.70582  SampleTime=0
  escalon2 : Step  Time=7.5  After=-0.70582  SampleTime=0
  esca : Outport
  wires:
  escalon2/1 -> Sum/2
  escalon1/1 -> Sum/1
  Sum/1 -> [esca], Scope3/1
  [esca] -> esca/1

== system controlGPI_pos_2dof_sinMI/Perfil torque de carga tau_L/If Action Subsystem3 ==
  Action Port : ActionPort
  Scope2 : Scope
  Sum2 : Sum  Inputs=|++
  rampa1 : simulink/Sources/Ramp  slope=0.02064  start=2.5  InitialOutput=0
  rampa2 : simulink/Sources/Ramp  slope=-0.02064  start=7.5  InitialOutput=0
  ramp : Outport
  wires:
  rampa2/1 -> Sum2/2
  rampa1/1 -> Sum2/1
  Sum2/1 -> Scope2/1, [ramp]
  [ramp] -> ramp/1

== system controlGPI_pos_2dof_sinMI/Perfil torque de carga tau_L/If Action Subsystem4 ==
  perfil_params : Inport
  Action Port : ActionPort
  Clock1 : Clock
  Polinomio 7mo orden tau_L : MATLAB Function  TreatAsAtomicUnit=on
  Scope : Scope  NumInputPorts=4
  pol7 : Outport
  wires:
  Polinomio 7mo orden tau_L/4(jpol) -> Scope/4
  Polinomio 7mo orden tau_L/1(qpol) -> Scope/1, [pol7]
  Polinomio 7mo orden tau_L/2(vpol) -> Scope/2
  Clock1/1 -> Polinomio 7mo orden tau_L/1(t)
  Polinomio 7mo orden tau_L/3(apol) -> Scope/3
  perfil_params/1 -> Polinomio 7mo orden tau_L/2(perfil_params)
  [pol7] -> pol7/1

== system controlGPI_pos_2dof_sinMI/Perfil torque de carga tau_L/If Action Subsystem5 ==
  perfil_params : Inport
  Action Port : ActionPort
  Clock : Clock
  Scope1 : Scope
  Tren de esca : MATLAB Function  TreatAsAtomicUnit=on
  trEsca : Outport
  wires:
  Tren de esca/1(q) -> Scope1/1, [trEsca]
  Clock/1 -> Tren de esca/1(t)
  perfil_params/1 -> Tren de esca/2(perfil_params)
  [trEsca] -> trEsca/1

== system controlGPI_pos_2dof_sinMI/Perfil torque de carga tau_L/If Action Subsystem6 ==
  Action Port : ActionPort
  Clock3 : Clock
  Polinomio 7mo orden timeseries : MATLAB Function  TreatAsAtomicUnit=on
  Product : Product
  Scope6 : Scope  NumInputPorts=4
  ts_data1 : FromWorkspace  Commented=on  VariableName=tau_L_ts
  ts : Outport
  wires:
  Product/1 -> [ts]
  Clock3/1 -> Polinomio 7mo orden timeseries/1(t)
  ts_data1/1 -> Product/1
  Polinomio 7mo orden timeseries/4(jpol) -> Scope6/4
  Polinomio 7mo orden timeseries/2(vpol) -> Scope6/2
  Polinomio 7mo orden timeseries/3(apol) -> Scope6/3
  Polinomio 7mo orden timeseries/1(qpol) -> Product/2, Scope6/1
  [ts] -> ts/1

== system controlGPI_pos_2dof_sinMI/Perfil torque de carga tau_L/If Action Subsystem7 ==
  perfil_params : Inport
  Action Port : ActionPort
  Clock5 : Clock
  Scope7 : Scope
  Trayectoria 15 segmentos : MATLAB Function  TreatAsAtomicUnit=on
  tr15segs : Outport
  wires:
  Clock5/1 -> Trayectoria 15 segmentos/1(t)
  Trayectoria 15 segmentos/1(q) -> Scope7/1, [tr15segs]
  [tr15segs] -> tr15segs/1
  perfil_params/1 -> Trayectoria 15 segmentos/2(perfil_params)

== system controlGPI_pos_2dof_sinMI/Trayectoria de referencia/2 to 2 (2) ==
  In1 : Inport
  In2 : Inport  Port=2
  Demux3 : Demux  Outputs=2
  Demux4 : Demux  Outputs=2
  Mux8 : Mux  Inputs=2
  Mux9 : Mux  Inputs=2
  1 : Outport
  2 : Outport  Port=2
  wires:
  Demux3/1 -> Mux8/1
  Demux3/2 -> Mux9/1
  Mux9/1 -> 2/1
  Demux4/2 -> Mux9/2
  Demux4/1 -> Mux8/2
  Mux8/1 -> 1/1
  In1/1 -> Demux3/1
  In2/1 -> Demux4/1

== system controlGPI_pos_2dof_sinMI/Trayectoria de referencia/2 to 2 (2)1 ==
  In1 : Inport
  In2 : Inport  Port=2
  Demux3 : Demux  Outputs=2
  Demux4 : Demux  Outputs=2
  Mux8 : Mux  Inputs=2
  Mux9 : Mux  Inputs=2
  1 : Outport
  2 : Outport  Port=2
  wires:
  Demux3/1 -> Mux8/1
  Demux3/2 -> Mux9/1
  Mux9/1 -> 2/1
  Demux4/2 -> Mux9/2
  Demux4/1 -> Mux8/2
  Mux8/1 -> 1/1
  In1/1 -> Demux3/1
  In2/1 -> Demux4/1

== system controlGPI_pos_2dof_sinMI/Trayectoria de referencia/2 to 2 (2)2 ==
  In1 : Inport
  In2 : Inport  Port=2
  Demux3 : Demux  Outputs=2
  Demux4 : Demux  Outputs=2
  Mux8 : Mux  Inputs=2
  Mux9 : Mux  Inputs=2
  1 : Outport
  2 : Outport  Port=2
  wires:
  Demux3/1 -> Mux8/1
  Demux3/2 -> Mux9/1
  Mux9/1 -> 2/1
  Demux4/2 -> Mux9/2
  Demux4/1 -> Mux8/2
  Mux8/1 -> 1/1
  In1/1 -> Demux3/1
  In2/1 -> Demux4/1

== system controlGPI_pos_2dof_sinMI/Trayectoria de referencia/3 to 6 (4) ==
  In1 : Inport
  In2 : Inport  Port=2
  In3 : Inport  Port=3
  Demux2 : Demux  Outputs=2
  Demux3 : Demux  Outputs=2
  Demux4 : Demux  Outputs=2
  Out1 : Outport
  Out2 : Outport  Port=2
  Out3 : Outport  Port=3
  Out4 : Outport  Port=4
  Out5 : Outport  Port=5
  Out6 : Outport  Port=6
  wires:
  In3/1 -> Demux4/1
  Demux4/1 -> Out3/1
  Demux2/1 -> Out1/1
  Demux3/2 -> Out5/1
  Demux3/1 -> Out2/1
  In1/1 -> Demux2/1
  Demux4/2 -> Out6/1
  Demux2/2 -> Out4/1
  In2/1 -> Demux3/1

== system controlGPI_pos_2dof_sinMI/Trayectoria de referencia/3 to 6 (4)1 ==
  In1 : Inport
  In2 : Inport  Port=2
  In3 : Inport  Port=3
  Demux2 : Demux  Outputs=2
  Demux3 : Demux  Outputs=2
  Demux4 : Demux  Outputs=2
  Out1 : Outport
  Out2 : Outport  Port=2
  Out3 : Outport  Port=3
  Out4 : Outport  Port=4
  Out5 : Outport  Port=5
  Out6 : Outport  Port=6
  wires:
  In3/1 -> Demux4/1
  Demux4/1 -> Out3/1
  Demux2/1 -> Out1/1
  Demux3/2 -> Out5/1
  Demux3/1 -> Out2/1
  In1/1 -> Demux2/1
  Demux4/2 -> Out6/1
  Demux2/2 -> Out4/1
  In2/1 -> Demux3/1

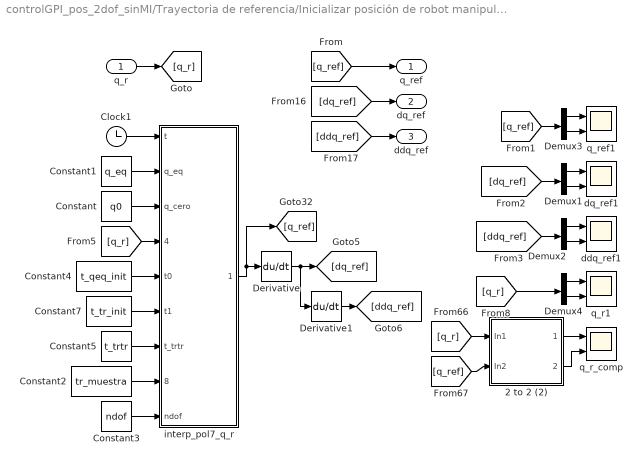
== system controlGPI_pos_2dof_sinMI/Trayectoria de referencia/Inicializar posición de robot manipulador ==
  q_r : Inport
  2 to 2 (2) : Subsystem
  Clock1 : Clock
  Constant : Constant  Value=q0
  Constant1 : Constant  Value=q_eq
  Constant2 : Constant  Value=tr_muestra
  Constant3 : Constant  Value=ndof
  Constant4 : Constant  Value=t_qeq_init
  Constant5 : Constant  Value=t_trtr
  Constant7 : Constant  Value=t_tr_init
  Demux{1..4} (4 alike) : Demux  Outputs=2
  Derivative : Derivative
  Derivative1 : Derivative
  ddq_ref1 : Scope  NumInputPorts=2
  dq_ref1 : Scope  NumInputPorts=2
  interp_pol7_q_r : MATLAB Function  TreatAsAtomicUnit=on
  q_r1 : Scope  NumInputPorts=2
  q_r_comp : Scope  NumInputPorts=2
  q_ref1 : Scope  NumInputPorts=2
  q_ref : Outport
  dq_ref : Outport  Port=2
  ddq_ref : Outport  Port=3
  wires:
  [ddq_ref] -> ddq_ref/1
  q_r/1 -> [q_r]
  [dq_ref] -> dq_ref/1
  [q_ref] -> q_ref/1
  [q_r] -> 2 to 2 (2)/1(In1)
  [q_ref] -> 2 to 2 (2)/2(In2)
  [q_r] -> Demux4/1
  interp_pol7_q_r/1(interp_qpos) -> [q_ref], Derivative/1
  Derivative/1 -> [dq_ref], Derivative1/1
  Derivative1/1 -> [ddq_ref]
  [q_ref] -> Demux3/1
  [dq_ref] -> Demux1/1
  [ddq_ref] -> Demux2/1
  Constant5/1 -> interp_pol7_q_r/7(t_trtr)
  Constant4/1 -> interp_pol7_q_r/5(t0)
  Constant1/1 -> interp_pol7_q_r/2(q_eq)
  [q_r] -> interp_pol7_q_r/4(q_tr_init)
  Constant3/1 -> interp_pol7_q_r/9(ndof)
  Constant/1 -> interp_pol7_q_r/3(q_cero)
  Clock1/1 -> interp_pol7_q_r/1(t)
  Constant7/1 -> interp_pol7_q_r/6(t1)
  Constant2/1 -> interp_pol7_q_r/8(tr_muestra)
  Demux3/1 -> q_ref1/1
  Demux3/2 -> q_ref1/2
  Demux1/1 -> dq_ref1/1
  Demux1/2 -> dq_ref1/2
  Demux2/1 -> ddq_ref1/1
  Demux2/2 -> ddq_ref1/2
  Demux4/1 -> q_r1/1
  Demux4/2 -> q_r1/2
  2 to 2 (2)/1(1) -> q_r_comp/1
  2 to 2 (2)/2(2) -> q_r_comp/2

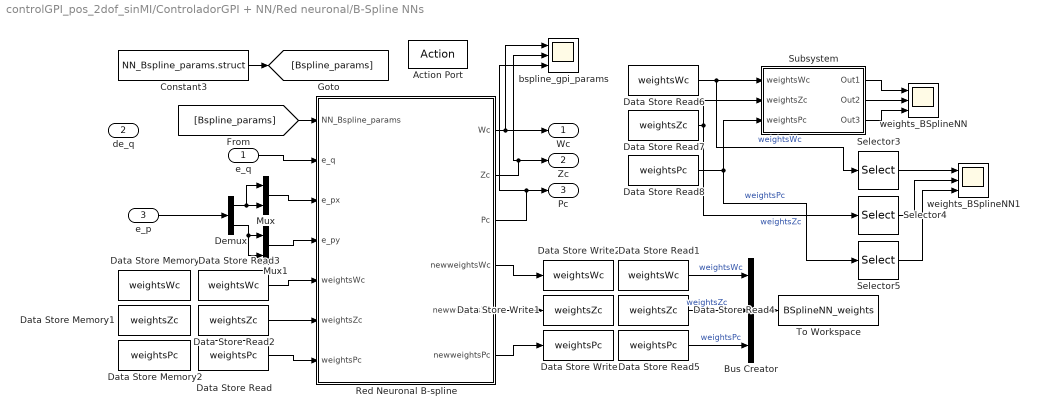
== system controlGPI_pos_2dof_sinMI/ControladorGPI + NN/Red neuronal/B-Spline NNs ==
  e_q : Inport
  de_q : Inport  Port=2
  e_p : Inport  Port=3
  Action Port : ActionPort  ActionPortLabel=if(u1 == 1)
  Bus Creator : BusCreator  Inputs=3
  Constant3 : Constant  Value=NN_Bspline_params.struct  OutDataTypeStr=Bus: NN_Bspline_params_bus
  Data Store Memory : DataStoreMemory  DataStoreName=weightsWc  WriteAfterWriteMsg=warning  InitialValue=NN_Bspline_params.weights.weightWc  ShowAdditionalParam=off  OutDataTypeStr=double
  Data Store Memory1 : DataStoreMemory  DataStoreName=weightsZc  WriteAfterWriteMsg=warning  InitialValue=NN_Bspline_params.weights.weightZc  ShowAdditionalParam=off  OutDataTypeStr=double
  Data Store Memory2 : DataStoreMemory  DataStoreName=weightsPc  WriteAfterWriteMsg=warning  InitialValue=NN_Bspline_params.weights.weightPc  ShowAdditionalParam=off  OutDataTypeStr=double
  Data Store Read : DataStoreRead  DataStoreName=weightsPc  IndexOptions=Index vector (dialog)  Indices=1  OutputSizes=1
  Data Store Read1 : DataStoreRead  DataStoreName=weightsWc  IndexOptions=Index vector (dialog)  Indices=1  OutputSizes=1
  Data Store Read2 : DataStoreRead  DataStoreName=weightsZc  IndexOptions=Index vector (dialog)  Indices=1  OutputSizes=1
  Data Store Read3 : DataStoreRead  DataStoreName=weightsWc  IndexOptions=Index vector (dialog)  Indices=1  OutputSizes=1
  Data Store Read4 : DataStoreRead  DataStoreName=weightsZc  IndexOptions=Index vector (dialog)  Indices=1  OutputSizes=1
  Data Store Read5 : DataStoreRead  DataStoreName=weightsPc  IndexOptions=Index vector (dialog)  Indices=1  OutputSizes=1
  Data Store Read6 : DataStoreRead  DataStoreName=weightsWc  IndexOptions=Index vector (dialog)  Indices=1  OutputSizes=1
  Data Store Read7 : DataStoreRead  DataStoreName=weightsZc  IndexOptions=Index vector (dialog)  Indices=1  OutputSizes=1
  Data Store Read8 : DataStoreRead  DataStoreName=weightsPc  IndexOptions=Index vector (dialog)  Indices=1  OutputSizes=1
  Data Store Write : DataStoreWrite  DataStoreName=weightsPc  IndexOptions=Index vector (dialog)  Indices=1  OutputSizes=1
  Data Store Write1 : DataStoreWrite  DataStoreName=weightsZc  IndexOptions=Index vector (dialog)  Indices=1  OutputSizes=1
  Data Store Write2 : DataStoreWrite  DataStoreName=weightsWc  IndexOptions=Index vector (dialog)  Indices=1  OutputSizes=1
  Demux : Demux  Outputs=2
  Mux : Mux  Inputs=2
  Mux1 : Mux  Inputs=2
  Red Neuronal B-spline : MATLAB Function  TreatAsAtomicUnit=on
  Selector3 : Selector  NumberOfDimensions=3  InputPortWidth=3  IndexOptions=Index vector (dialog),Index vector (dialog),Index vector (dialog)  Indices=1,[1:3],2  OutputSizes=1,1,1
  Selector4 : Selector  NumberOfDimensions=3  InputPortWidth=3  IndexOptions=Index vector (dialog),Index vector (dialog),Index vector (dialog)  Indices=1,[1:3],2  OutputSizes=1,1,1
  Selector5 : Selector  NumberOfDimensions=3  InputPortWidth=3  IndexOptions=Index vector (dialog),Index vector (dialog),Index vector (dialog)  Indices=1,[1:3],2  OutputSizes=1,1,1
  Subsystem : Subsystem
  To Workspace : ToWorkspace  VariableName=BSplineNN_weights  SaveFormat=Timeseries  SampleTime=-1
  bspline_gpi_params : Scope  NumInputPorts=3
  weights_BSplineNN : Scope  NumInputPorts=3
  weights_BSplineNN1 : Scope  NumInputPorts=3
  Wc : Outport
  Zc : Outport  Port=2
  Pc : Outport  Port=3
  wires:
  e_q/1 -> Red Neuronal B-spline/2(e_q)
  [Bspline_params] -> Red Neuronal B-spline/1(NN_Bspline_params)
  Red Neuronal B-spline/1(Wc) -> Wc/1, bspline_gpi_params/1
  Red Neuronal B-spline/2(Zc) -> bspline_gpi_params/2, Zc/1
  Red Neuronal B-spline/3(Pc) -> bspline_gpi_params/3, Pc/1
  Constant3/1 -> [Bspline_params]
  Data Store Read1/1 -> Bus Creator/1  "weightsWc"
  Data Store Read5/1 -> Bus Creator/3  "weightsPc"
  Bus Creator/1 -> To Workspace/1
  Data Store Read4/1 -> Bus Creator/2  "weightsZc"
  Red Neuronal B-spline/4(newweightsWc) -> Data Store Write2/1
  Red Neuronal B-spline/5(newweightsZc) -> Data Store Write1/1
  Red Neuronal B-spline/6(newweightsPc) -> Data Store Write/1
  Data Store Read3/1 -> Red Neuronal B-spline/5(weightsWc)
  Data Store Read2/1 -> Red Neuronal B-spline/6(weightsZc)
  Data Store Read/1 -> Red Neuronal B-spline/7(weightsPc)
  Demux/2 -> Mux1/2, Mux1/1
  e_p/1 -> Demux/1
  Demux/1 -> Mux/1, Mux/2
  Mux/1 -> Red Neuronal B-spline/3(e_px)
  Mux1/1 -> Red Neuronal B-spline/4(e_py)
  Data Store Read6/1 -> Selector3/1, Subsystem/1(weightsWc)  "weightsWc"
  Data Store Read7/1 -> Subsystem/2(weightsZc), Selector4/1  "weightsZc"
  Data Store Read8/1 -> Selector5/1, Subsystem/3(weightsPc)  "weightsPc"
  Selector3/1 -> weights_BSplineNN1/1
  Selector4/1 -> weights_BSplineNN1/2
  Selector5/1 -> weights_BSplineNN1/3
  Subsystem/1(Out1) -> weights_BSplineNN/1
  Subsystem/2(Out2) -> weights_BSplineNN/2
  Subsystem/3(Out3) -> weights_BSplineNN/3

== system controlGPI_pos_2dof_sinMI/ControladorGPI + NN/Red neuronal/Constants ==
  Action Port : ActionPort  ActionPortLabel=else
  Constant : Constant  Value=Wc
  Constant1 : Constant  Value=Zc
  Constant2 : Constant  Value=Pc
  Scope1 : Scope  NumInputPorts=3
  Wc : Outport
  Zc : Outport  Port=2
  Pc : Outport  Port=3
  wires:
  Constant/1 -> Wc/1, Scope1/1
  Constant2/1 -> Scope1/3, Pc/1
  Constant1/1 -> Zc/1, Scope1/2

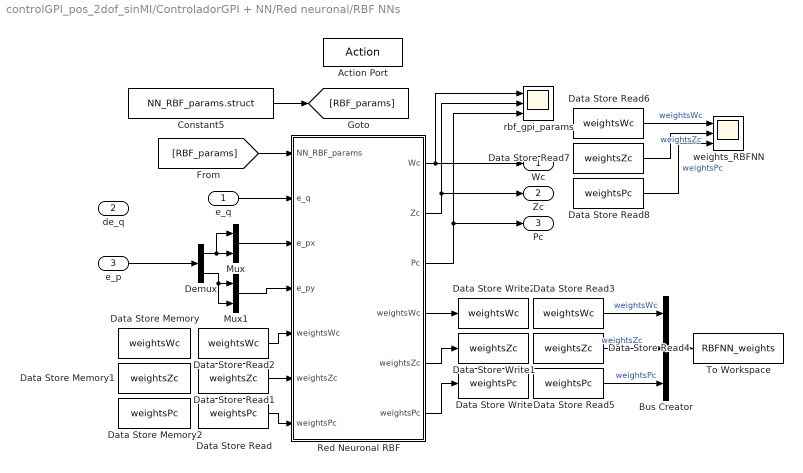
== system controlGPI_pos_2dof_sinMI/ControladorGPI + NN/Red neuronal/RBF NNs ==
  e_q : Inport
  de_q : Inport  Port=2
  e_p : Inport  Port=3
  Action Port : ActionPort  ActionPortLabel=elseif(u1 == 2)
  Bus Creator : BusCreator  Inputs=3
  Constant5 : Constant  Value=NN_RBF_params.struct  OutDataTypeStr=Bus: NN_RBF_params_bus
  Data Store Memory : DataStoreMemory  DataStoreName=weightsWc  WriteAfterWriteMsg=warning  InitialValue=NN_RBF_params.weights.weightWc  ShowAdditionalParam=off  OutDataTypeStr=double
  Data Store Memory1 : DataStoreMemory  DataStoreName=weightsZc  WriteAfterWriteMsg=warning  InitialValue=NN_RBF_params.weights.weightZc  ShowAdditionalParam=off  OutDataTypeStr=double
  Data Store Memory2 : DataStoreMemory  DataStoreName=weightsPc  WriteAfterWriteMsg=warning  InitialValue=NN_RBF_params.weights.weightPc  ShowAdditionalParam=off  OutDataTypeStr=double
  Data Store Read : DataStoreRead  DataStoreName=weightsPc  IndexOptions=Index vector (dialog)  Indices=1  OutputSizes=1
  Data Store Read1 : DataStoreRead  DataStoreName=weightsZc  IndexOptions=Index vector (dialog)  Indices=1  OutputSizes=1
  Data Store Read2 : DataStoreRead  DataStoreName=weightsWc  IndexOptions=Index vector (dialog)  Indices=1  OutputSizes=1
  Data Store Read3 : DataStoreRead  DataStoreName=weightsWc  IndexOptions=Index vector (dialog)  Indices=1  OutputSizes=1
  Data Store Read4 : DataStoreRead  DataStoreName=weightsZc  IndexOptions=Index vector (dialog)  Indices=1  OutputSizes=1
  Data Store Read5 : DataStoreRead  DataStoreName=weightsPc  IndexOptions=Index vector (dialog)  Indices=1  OutputSizes=1
  Data Store Read6 : DataStoreRead  DataStoreName=weightsWc  IndexOptions=Index vector (dialog)  Indices=1  OutputSizes=1
  Data Store Read7 : DataStoreRead  DataStoreName=weightsZc  IndexOptions=Index vector (dialog)  Indices=1  OutputSizes=1
  Data Store Read8 : DataStoreRead  DataStoreName=weightsPc  IndexOptions=Index vector (dialog)  Indices=1  OutputSizes=1
  Data Store Write : DataStoreWrite  DataStoreName=weightsPc  IndexOptions=Index vector (dialog)  Indices=1  OutputSizes=1
  Data Store Write1 : DataStoreWrite  DataStoreName=weightsZc  IndexOptions=Index vector (dialog)  Indices=1  OutputSizes=1
  Data Store Write2 : DataStoreWrite  DataStoreName=weightsWc  IndexOptions=Index vector (dialog)  Indices=1  OutputSizes=1
  Demux : Demux  Outputs=2
  Mux : Mux  Inputs=2
  Mux1 : Mux  Inputs=2
  Red Neuronal RBF : MATLAB Function  TreatAsAtomicUnit=on
  To Workspace : ToWorkspace  VariableName=RBFNN_weights  SaveFormat=Timeseries  SampleTime=-1
  rbf_gpi_params : Scope  NumInputPorts=3
  weights_RBFNN : Scope  NumInputPorts=3
  Wc : Outport
  Zc : Outport  Port=2
  Pc : Outport  Port=3
  wires:
  [RBF_params] -> Red Neuronal RBF/1(NN_RBF_params)
  e_q/1 -> Red Neuronal RBF/2(e_q)
  Red Neuronal RBF/1(Wc) -> rbf_gpi_params/1, Wc/1
  Red Neuronal RBF/2(Zc) -> rbf_gpi_params/2, Zc/1
  Red Neuronal RBF/3(Pc) -> rbf_gpi_params/3, Pc/1
  Data Store Read/1 -> Red Neuronal RBF/7("weightsPc ")
  Data Store Read1/1 -> Red Neuronal RBF/6("weightsZc ")
  Data Store Read2/1 -> Red Neuronal RBF/5("weightsWc ")
  Data Store Read3/1 -> Bus Creator/1  "weightsWc"
  Data Store Read4/1 -> Bus Creator/2  "weightsZc"
  Data Store Read5/1 -> Bus Creator/3  "weightsPc"
  Bus Creator/1 -> To Workspace/1
  Red Neuronal RBF/6(weightsPc) -> Data Store Write/1
  Red Neuronal RBF/4(weightsWc) -> Data Store Write2/1
  Red Neuronal RBF/5(weightsZc) -> Data Store Write1/1
  Data Store Read6/1 -> weights_RBFNN/1  "weightsWc"
  Data Store Read7/1 -> weights_RBFNN/2  "weightsZc"
  Data Store Read8/1 -> weights_RBFNN/3  "weightsPc"
  Constant5/1 -> [RBF_params]
  e_p/1 -> Demux/1
  Mux/1 -> Red Neuronal RBF/3(e_px)
  Demux/1 -> Mux/1, Mux/2
  Demux/2 -> Mux1/2, Mux1/1
  Mux1/1 -> Red Neuronal RBF/4(e_py)

== system controlGPI_pos_2dof_sinMI/Trayectoria de referencia/Inicializar posición de robot manipulador/2 to 2 (2) ==
  In1 : Inport
  In2 : Inport  Port=2
  Demux3 : Demux  Outputs=2
  Demux4 : Demux  Outputs=2
  Mux8 : Mux  Inputs=2
  Mux9 : Mux  Inputs=2
  1 : Outport
  2 : Outport  Port=2
  wires:
  Demux3/1 -> Mux8/1
  Demux3/2 -> Mux9/1
  Mux9/1 -> 2/1
  Demux4/2 -> Mux9/2
  Demux4/1 -> Mux8/2
  Mux8/1 -> 1/1
  In1/1 -> Demux3/1
  In2/1 -> Demux4/1

== system controlGPI_pos_2dof_sinMI/ControladorGPI + NN/Red neuronal/B-Spline NNs/Subsystem ==
  weightsWc : Inport
  weightsZc : Inport  Port=2
  weightsPc : Inport  Port=3
  Selector : Selector  NumberOfDimensions=3  InputPortWidth=3  IndexOptions=Index vector (dialog),Index vector (dialog),Index vector (dialog)  Indices=1,[1:3],2  OutputSizes=1,1,1
  Selector1 : Selector  NumberOfDimensions=3  InputPortWidth=3  IndexOptions=Index vector (dialog),Index vector (dialog),Index vector (dialog)  Indices=1,[1:3],1  OutputSizes=1,1,1
  Selector2 : Selector  NumberOfDimensions=3  InputPortWidth=3  IndexOptions=Index vector (dialog),Index vector (dialog),Index vector (dialog)  Indices=1,[1:3],1  OutputSizes=1,1,1
  Out1 : Outport
  Out2 : Outport  Port=2
  Out3 : Outport  Port=3
  wires:
  weightsZc/1 -> Selector1/1
  weightsPc/1 -> Selector2/1
  weightsWc/1 -> Selector/1
  Selector1/1 -> Out2/1
  Selector2/1 -> Out3/1
  Selector/1 -> Out1/1

== matlab function controlGPI_pos_2dof_sinMI/Trayectoria de referencia/xyz to q (referencia) ==
  data: robot_params input; q output size=[2,1]; r input size=[2,1]; dr input size=[2,1]; ddr input size=[2,1]; dq output size=[2,1]; ddq output size=[2,1]
function [q,dq,ddq] = fcn(robot_params,r,dr,ddr)

[q,dq,ddq] = robot_cin.cin_inv_2dof(robot_params,r,dr,ddr);

== matlab function controlGPI_pos_2dof_sinMI/ControladorGPI + NN/Matriz D ==
  data: robot_params input Bus: robot_params_bus; robot_din output Bus: robot_din_bus; q input
function robot_din = fcn(robot_params,q)

robot_din = robot_dinm.din_2dof(robot_params,q,zeros(size(q)));

== matlab function controlGPI_pos_2dof_sinMI/Perfil torque de carga tau_L/If Action Subsystem/Polinomio 7mo orden sen ==
  data: t input; perfil_params input; qpol output; vpol output; apol output; jpol output
function [qpol,vpol,apol,jpol] = fcn(t,perfil_params)

%Trayectoria de referencia

q0 = 0;
q1 = perfil_params.senoidal.amplitud;

% v0 = perfil_params.polinomio7.vel.inicial;
% v1 = perfil_params.polinomio7.vel.final;
% 
% ac0 = perfil_params.polinomio7.acel.inicial;
% ac1 = perfil_params.polinomio7.acel.final;
% 
% j0 = perfil_params.polinomio7.jerk.inicial;
% j1 = perfil_params.polinomio7.jerk.inicial;

if perfil_params.senoidal.tiempo_inicio-1>0
    t0 = perfil_params.senoidal.tiempo_inicio-1;
else
    t0 = 0;
end
t1 = perfil_params.senoidal.tiempo_inicio;

% Coeficientes de un polinomio de 7mo grado
[qpol,vpol,apol,jpol] = pol7(t,q1,q0,t0,t1);

== matlab function controlGPI_pos_2dof_sinMI/Perfil torque de carga tau_L/If Action Subsystem4/Polinomio 7mo orden tau_L ==
  data: t input; perfil_params input; qpol output; vpol output; apol output; jpol output
function [qpol,vpol,apol,jpol] = fcn(t,perfil_params)

%Trayectoria de referencia

q0 = perfil_params.polinomio7.pos.inicial;
q1 = perfil_params.polinomio7.pos.final;

% v0 = perfil_params.polinomio7.vel.inicial;
% v1 = perfil_params.polinomio7.vel.final;
% 
% ac0 = perfil_params.polinomio7.acel.inicial;
% ac1 = perfil_params.polinomio7.acel.final;
% 
% j0 = perfil_params.polinomio7.jerk.inicial;
% j1 = perfil_params.polinomio7.jerk.inicial;

t0 = perfil_params.polinomio7.tiempo.inicial;
t1 = perfil_params.polinomio7.tiempo.final;

% Coeficientes de un polinomio de 7mo grado
[qpol,vpol,apol,jpol] = pol7(t,q0,q1,t0,t1);

== matlab function controlGPI_pos_2dof_sinMI/Perfil torque de carga tau_L/If Action Subsystem7/Trayectoria 15 segmentos ==
  data: t input size=1; q output size=1; perfil_params input
function q = fcn(t,perfil_params)

q0 = perfil_params.tr15segs.pos.inicial;
q1 = perfil_params.tr15segs.pos.final;

t0 = perfil_params.tr15segs.tiempo.inicial;

vel_path = perfil_params.tr15segs.vel_path;
acel_path = perfil_params.tr15segs.acel_path;
snap_path = perfil_params.tr15segs.snap_path;

dist = norm(q1-q0);
num_steps = 1000;




[interq,T] = pol15segs.bounded_tr(dist,num_steps,vel_path,acel_path,snap_path,0);

tstep = T/num_steps;
t1 = t0 + T;
t_tr = (t0:tstep:t1)';


[~,idt] = min(t_tr-t);
dire = (q1 - q0)/dist;
q = q0 + dire*interq(idt);

== matlab function controlGPI_pos_2dof_sinMI/Perfil torque de carga tau_L/If Action Subsystem6/Polinomio 7mo orden timeseries ==
  data: t input; qpol output; vpol output; apol output; jpol output
function [qpol,vpol,apol,jpol] = fcn(t)

q0 = 0;
q1 = 1;

t0 = 0.5;
t1 = 1;

%Trayectoria de referencia

% Coeficientes de un polinomio de 7mo grado
[qpol,vpol,apol,jpol] = pol7(t,q0,q1,t0,t1);

== matlab function controlGPI_pos_2dof_sinMI/Perfil torque de carga tau_L/If Action Subsystem/Senoidal tiempo de inicio ==
  data: t input; tr output; perfil_params input
function tr = fcn(t,perfil_params)

t1 = perfil_params.senoidal.tiempo_inicio;

if t < t1
    tr = 0;
else
    tr = t - t1;
end

== matlab function controlGPI_pos_2dof_sinMI/Perfil torque de carga tau_L/If Action Subsystem5/Tren de esca ==
  data: t input; q output; perfil_params input
function q = fcn(t,perfil_params)

q = Perfil_trayectoria.trEsca(t,perfil_params);

== matlab function controlGPI_pos_2dof_sinMI/Modelo robot manipulador (Dinámica directa)/Dinámica directa ==
  data: robot_params input; q input; ddq output size=[2,1]; dq input size=[2,1]; tau_R input size=[2,1]; tau_L input size=[2,1]
function ddq = fcn(robot_params,q,dq,tau_R,tau_L)

robot_din = robot_dinm.din_2dof(robot_params,q,dq);

D = robot_din.D;
C = robot_din.C;
G = robot_din.G;
g = robot_din.g;

ddq = D^-1*(-C*dq-G*g+(tau_R-tau_L));
